simulink model "estimate_battery_soca"  (R2022a)
settings: Solver=VariableStepAuto  StartTime=0.0  StopTime=t_end  RelTol=1e-3
undefined symbols (not defined in the file): Bat_cap, eff_bcr, eff_id, eff_pcm, Np, Ns, OCV, Ri_cell, sigbuilder_block, SOC, SOC_init, V_ulim
settings Model: Creator=Geuk-Nam Kim  LastModifiedBy=ACL2022_13
settings SolverCC: ZeroCrossAlgorithm=Adaptive  AlgebraicLoopSolver=TrustRegion
settings DebuggingCC: IgnoredZcDiagnostic=none  UnconnectedInputMsg=warning  UnconnectedOutputMsg=warning  UnconnectedLineMsg=warning  SFMachineParentedDataDiag=warning

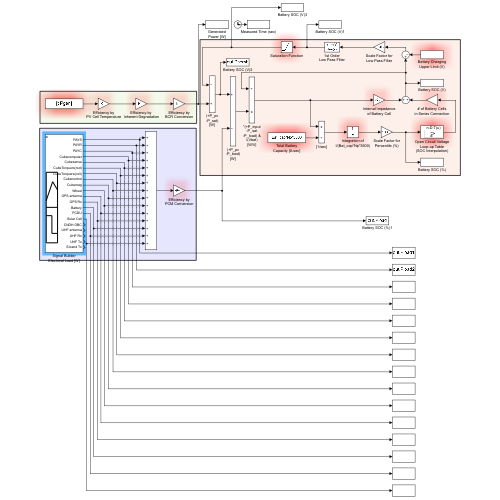
[thumbnail: Simulink's stored preview of the top-level diagram]
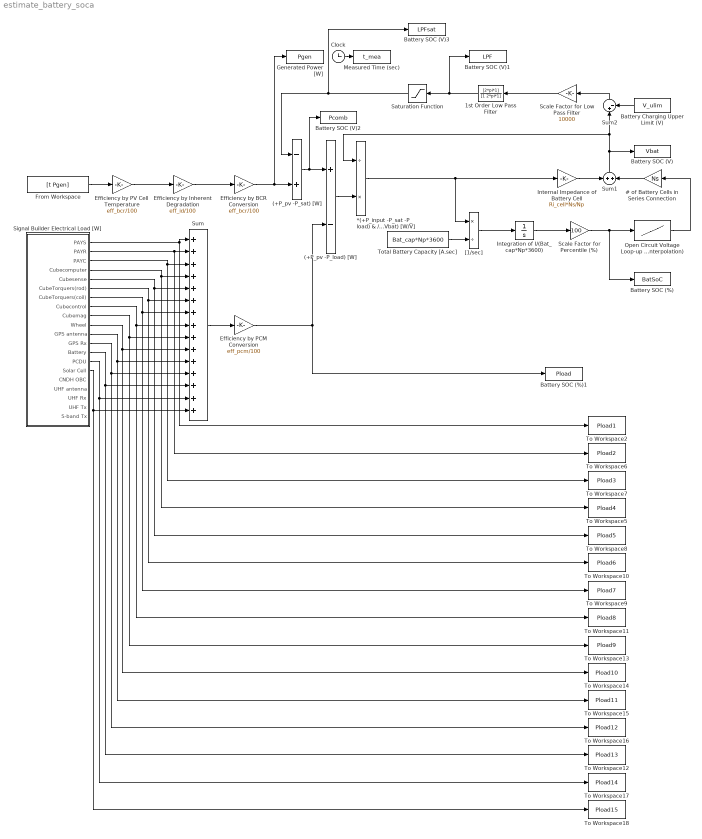
== system estimate_battery_soca ==
  # of Battery Cells in Series Connection : Gain  Gain=Ns
  (+P_pv -P_load) [W] : Sum  Inputs=+-
  (+P_pv -P_sat) [W] : Sum  Inputs=-+
  *(+P_input -P_sat -P_load) & /(Vbat) [W/V] : Product  Inputs=/*
  1st Order Low Pass Filter : TransferFcn  Numerator=[2*pi*1]  Denominator=[1 2*pi*1]
  Battery Charging Upper Limit (V) : Constant  Value=V_ulim
  Battery SOC (%) : ToWorkspace  VariableName=BatSoC  SampleTime=-1
  Battery SOC (%)1 : ToWorkspace  VariableName=Pload  SampleTime=-1
  Battery SOC (V) : ToWorkspace  VariableName=Vbat  SampleTime=-1
  Battery SOC (V)1 : ToWorkspace  VariableName=LPF  SampleTime=-1
  Battery SOC (V)2 : ToWorkspace  VariableName=Pcomb  SampleTime=-1
  Battery SOC (V)3 : ToWorkspace  VariableName=LPFsat  SampleTime=-1
  Clock : Clock
  "Efficiency by BCR Conversion " : Gain  Gain=eff_bcr/100
  Efficiency by PCM Conversion : Gain  Gain=eff_pcm/100
  Efficiency by PV Cell Temperature : Gain  Gain=eff_bcr/100
  Efficiency by Inherent Degradation : Gain  Gain=eff_id/100
  From Workspace : FromWorkspace  VariableName=[t Pgen]  SampleTime=-1
  Generated Power [W] : ToWorkspace  VariableName=Pgen  SampleTime=-1
  Integration of I/(Bat_cap*Np*3600) : Integrator  InitialCondition=SOC_init
  Internal Impedance of Battery Cell : Gain  Gain=Ri_cell*Ns/Np
  Measured Time (sec) : ToWorkspace  VariableName=t_mea  SampleTime=-1
  Open Circuit Voltage Loop-up Table (SOC Interpolation) : Lookup_n-D  NumberOfTableDimensions=1  BreakpointsForDimension1=SOC  Table=OCV  InternalRulePriority=Speed  RndMeth=Simplest
  Saturation Function : Saturate  UpperLimit=V_ulim  LowerLimit=0
  Scale Factor for Low Pass Filter : Gain  Gain=10000
  Scale Factor for Percentile (%) : Gain  Gain=100
  Signal Builder Electrical Load [W] : Subsystem  Tag=STV Subsys  LoadFcn=sigbuilder_block('load',[6 30 1428 680.25 ]);  StartFcn=sigbuilder_block('start');  StopFcn=sigbuilder_block('stop');  ClipboardFcn=sigbuilder_block('clipboard');  mask(Sigbuilder block){tuvar=[0:10]}
      mask help: Simulink:masks:SigbuilderBlock_MD
      mask init:
      | if ~strcmp(get_param(bdroot(gcbh),'SimulationStatus'),'stopped') tuvar = sigbuilder_block('maskInit'); end
      settings: CopyFcn=sigbuilder_block('copy');  DeleteFcn=sigbuilder_block('delete');  ModelCloseFcn=sigbuilder_block('modelClose');  PreSaveFcn=sigbuilder_block('preSave');  PauseFcn=sigbuilder_block('pause');  ContinueFcn=sigbuilder_block('continue');  NameChangeFcn=sigbuilder_block('namechange');  OpenFcn=sigbuilder_block('open',[6 30 1428 680.25 ]);  CloseFcn=sigbuilder_block('close');
      mask Display: plot(0, 0, 100, 100,[2, 2, 32, 32, 2], [68, 8, 8, 68, 68],[32, 2], [38, 38], [32, 19, 2],[53, 60, 44], [32, 17, 17, 2],[16, 16, 31, 31]);txt = getActiveGroup(gcbh);text(2, 100, txt,'verticalAlignment', 'top');
  Sum : Sum  Inputs=15
  Sum1 : Sum  Inputs=+|+
  Sum2 : Sum  Inputs=|+-
  To Workspace10 : ToWorkspace  VariableName=Pload6  SampleTime=-1
  To Workspace11 : ToWorkspace  VariableName=Pload8  SampleTime=-1
  To Workspace12 : ToWorkspace  VariableName=Pload13  SampleTime=-1
  To Workspace13 : ToWorkspace  VariableName=Pload9  SampleTime=-1
  To Workspace14 : ToWorkspace  VariableName=Pload10  SampleTime=-1
  To Workspace15 : ToWorkspace  VariableName=Pload11  SampleTime=-1
  To Workspace16 : ToWorkspace  VariableName=Pload12  SampleTime=-1
  To Workspace17 : ToWorkspace  VariableName=Pload14  SampleTime=-1
  To Workspace18 : ToWorkspace  VariableName=Pload15  SampleTime=-1
  To Workspace2 : ToWorkspace  VariableName=Pload1  SampleTime=-1
  To Workspace5 : ToWorkspace  VariableName=Pload4  SampleTime=-1
  To Workspace6 : ToWorkspace  VariableName=Pload2  SampleTime=-1
  To Workspace7 : ToWorkspace  VariableName=Pload3  SampleTime=-1
  To Workspace8 : ToWorkspace  VariableName=Pload5  SampleTime=-1
  To Workspace9 : ToWorkspace  VariableName=Pload7  SampleTime=-1
  Total Battery Capacity [A.sec] : Constant  Value=Bat_cap*Np*3600
  "[1/sec]" : Product  Inputs=*/
  wires:
  From Workspace/1 -> Efficiency by PV Cell Temperature/1
  Open Circuit Voltage Loop-up Table (SOC Interpolation)/1 -> # of Battery Cells in Series Connection/1
  Signal Builder Electrical Load [W]/8(Cubecontrol) -> To Workspace11/1, Sum/8
  Total Battery Capacity [A.sec]/1 -> "[1/sec]"/2
  Sum2/1 -> Scale Factor for Low Pass Filter/1
  "[1/sec]"/1 -> Integration of I/(Bat_cap*Np*3600)/1
  Scale Factor for Percentile (%)/1 -> Battery SOC (%)/1, Open Circuit Voltage Loop-up Table (SOC Interpolation)/1
  Signal Builder Electrical Load [W]/1(PAYS) -> Sum/1, To Workspace2/1
  "Efficiency by BCR Conversion "/1 -> (+P_pv -P_sat) [W]/2, Generated Power [W]/1
  Signal Builder Electrical Load [W]/14(PCDU) -> To Workspace17/1, Sum/14
  # of Battery Cells in Series Connection/1 -> Sum1/2
  Signal Builder Electrical Load [W]/4(Cubecomputer) -> To Workspace5/1, Sum/4
  Integration of I/(Bat_cap*Np*3600)/1 -> Scale Factor for Percentile (%)/1
  *(+P_input -P_sat -P_load) & /(Vbat) [W/V]/1 -> "[1/sec]"/1, Internal Impedance of Battery Cell/1
  Internal Impedance of Battery Cell/1 -> Sum1/1
  1st Order Low Pass Filter/1 -> Battery SOC (V)1/1, Saturation Function/1
  Signal Builder Electrical Load [W]/12(GPS Rx) -> To Workspace16/1, Sum/12
  Signal Builder Electrical Load [W]/13(Battery) -> To Workspace12/1, Sum/13
  Saturation Function/1 -> Battery SOC (V)3/1, (+P_pv -P_sat) [W]/1
  Signal Builder Electrical Load [W]/10(Wheel) -> To Workspace14/1, Sum/10
  (+P_pv -P_load) [W]/1 -> *(+P_input -P_sat -P_load) & /(Vbat) [W/V]/2
  Signal Builder Electrical Load [W]/11(GPS antenna) -> To Workspace15/1, Sum/11
  Signal Builder Electrical Load [W]/2(PAYR) -> To Workspace6/1, Sum/2
  Battery Charging Upper Limit (V)/1 -> Sum2/2
  Signal Builder Electrical Load [W]/15(Solar Cell) -> To Workspace18/1, Sum/15
  Signal Builder Electrical Load [W]/6(CubeTorquers(rod)) -> To Workspace10/1, Sum/6
  Sum1/1 -> Sum2/1, *(+P_input -P_sat -P_load) & /(Vbat) [W/V]/1, Battery SOC (V)/1
  Signal Builder Electrical Load [W]/5(Cubesense) -> To Workspace8/1, Sum/5
  Signal Builder Electrical Load [W]/9(Cubemag) -> To Workspace13/1, Sum/9
  Clock/1 -> Measured Time (sec)/1
  Efficiency by Inherent Degradation/1 -> "Efficiency by BCR Conversion "/1
  Sum/1 -> Efficiency by PCM Conversion/1
  Signal Builder Electrical Load [W]/3(PAYC) -> To Workspace7/1, Sum/3
  Efficiency by PV Cell Temperature/1 -> Efficiency by Inherent Degradation/1
  Signal Builder Electrical Load [W]/7(CubeTorquers(coil)) -> To Workspace9/1, Sum/7
  (+P_pv -P_sat) [W]/1 -> Battery SOC (V)2/1, (+P_pv -P_load) [W]/1
  Scale Factor for Low Pass Filter/1 -> 1st Order Low Pass Filter/1
  Efficiency by PCM Conversion/1 -> Battery SOC (%)1/1, (+P_pv -P_load) [W]/2

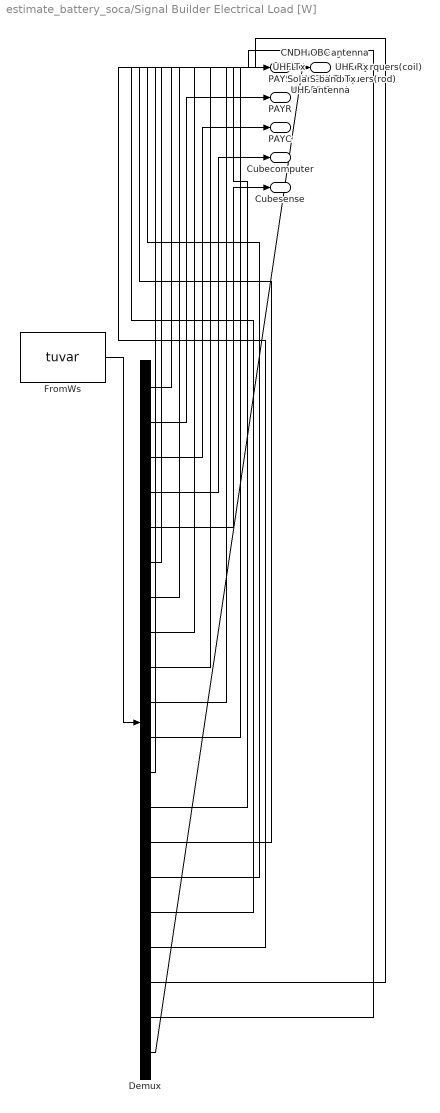
== system estimate_battery_soca/Signal Builder Electrical Load [W] ==
  Demux : Demux  Tag=STV Demux  Outputs=20
      settings: DisplayOption=none
  FromWs : FromWorkspace  Tag=STV FromWs  VariableName=tuvar
      SigBuilderData=|
      | common.afterFinalStr = 'Extrapolate'
      | common.sampleTime = '0'
      | dataSet(1).timeRange = [1 5678]
      | dataSet(1).name = 'a'
      | dataSet(2).timeRange = [1 5678]
      | dataSet(2).name = 'b'
      | dataSet(3).timeRange = [1 5678]
      | dataSet(3).name = 'c'
      | dataSet(4).timeRange = [1 5678]
      | dataSet(4).name = 'd'
      | sbobj.Name = 'Signal Builder'
      | sbobj.Groups(1).Name = 'a'
      | sbobj.Groups(1).Signals(1).Name = 'PAYS'
      | sbobj.Groups(1).Signals(1).XData = [1 2 3 4 5 6 7 8 9 10 11 12 ... (5678 elements, 1x5678)]
      | sbobj.Groups(1).Signals(1).YData = [0.2 0.2 0.2 0.2 0.2 0.2 0.2 0.2 0.2 0.2 0.2 0.2 ... (5678 elements, 1x5678)]
      | sbobj.Groups(1).Signals(2).Name = 'PAYR'
      | sbobj.Groups(1).Signals(2).XData = [1 2 3 4 5 6 7 8 9 10 11 12 ... (5678 elements, 1x5678)]
      | sbobj.Groups(1).Signals(2).YData = [0 0 0 0 0 0 0 0 0 0 0 0 ... (5678 elements, 1x5678)]
      | sbobj.Groups(1).Signals(3).Name = 'PAYC'
      | sbobj.Groups(1).Signals(3).XData = [1 2 3 4 5 6 7 8 9 10 11 12 ... (5678 elements, 1x5678)]
      | sbobj.Groups(1).Signals(3).YData = [1.3002 1.3002 1.3002 1.3002 1.3002 1.3002 1.3002 1.3002 1.3002 1.3002 1.3002 1.3002 ... (5678 elements, 1x5678)]
      | sbobj.Groups(1).Signals(4).Name = 'Cubecomputer'
      | sbobj.Groups(1).Signals(4).XData = [1 2 3 4 5 6 7 8 9 10 11 12 ... (5678 elements, 1x5678)]
      | sbobj.Groups(1).Signals(4).YData = [0.44 0.44 0.44 0.44 0.44 0.44 0.44 0.44 0.44 0.44 0.44 0.44 ... (5678 elements, 1x5678)]
      | sbobj.Groups(1).Signals(5).Name = 'Cubesense'
      | sbobj.Groups(1).Signals(5).XData = [1 2 3 4 5 6 7 8 9 10 11 12 ... (5678 elements, 1x5678)]
      | sbobj.Groups(1).Signals(5).YData = [0.8 0.8 0.8 0.8 0.8 0.8 0.8 0.8 0.8 0.8 0.8 0.8 ... (5678 elements, 1x5678)]
      | sbobj.Groups(1).Signals(6).Name = 'CubeTorquers(rod)'
      | sbobj.Groups(1).Signals(6).XData = [1 2 3 4 5 6 7 8 9 10 11 12 ... (5678 elements, 1x5678)]
      | sbobj.Groups(1).Signals(6).YData = [1.535 1.535 1.535 1.535 1.535 1.535 1.535 1.535 1.535 1.535 1.535 1.535 ... (5678 elements, 1x5678)]
      | sbobj.Groups(1).Signals(7).Name = 'CubeTorquers(coil)'
      | sbobj.Groups(1).Signals(7).XData = [1 2 3 4 5 6 7 8 9 10 11 12 ... (5678 elements, 1x5678)]
      | sbobj.Groups(1).Signals(7).YData = [0.192 0.192 0.192 0.192 0.192 0.192 0.192 0.192 0.192 0.192 0.192 0.192 ... (5678 elements, 1x5678)]
      | sbobj.Groups(1).Signals(8).Name = 'Cubecontrol'
      | sbobj.Groups(1).Signals(8).XData = [1 2 3 4 5 6 7 8 9 10 11 12 ... (5678 elements, 1x5678)]
      | sbobj.Groups(1).Signals(8).YData = [0.6 0.6 0.6 0.6 0.6 0.6 0.6 0.6 0.6 0.6 0.6 0.6 ... (5678 elements, 1x5678)]
      | sbobj.Groups(1).Signals(9).Name = 'Cubemag'
      | sbobj.Groups(1).Signals(9).XData = [1 2 3 4 5 6 7 8 9 10 11 12 ... (5678 elements, 1x5678)]
      | sbobj.Groups(1).Signals(9).YData = [0.105 0.105 0.105 0.105 0.105 0.105 0.105 0.105 0.105 0.105 0.105 0.105 ... (5678 elements, 1x5678)]
      | sbobj.Groups(1).Signals(10).Name = 'Wheel'
      | sbobj.Groups(1).Signals(10).XData = [1 2 3 4 5 6 7 8 9 10 11 12 ... (5678 elements, 1x5678)]
      | sbobj.Groups(1).Signals(10).YData = [8.04 8.04 8.04 8.04 8.04 8.04 8.04 8.04 8.04 8.04 8.04 8.04 ... (5678 elements, 1x5678)]
      | sbobj.Groups(1).Signals(11).Name = 'GPS antenna'
      | sbobj.Groups(1).Signals(11).XData = [1 2 3 4 5 6 7 8 9 10 11 12 ... (5678 elements, 1x5678)]
      | sbobj.Groups(1).Signals(11).YData = [0 0 0 0 0 0 0 0 0 0 0 0 ... (5678 elements, 1x5678)]
      | sbobj.Groups(1).Signals(12).Name = 'GPS Rx'
      | sbobj.Groups(1).Signals(12).XData = [1 2 3 4 5 6 7 8 9 10 11 12 ... (5678 elements, 1x5678)]
      | sbobj.Groups(1).Signals(12).YData = [3.9 3.9 3.9 3.9 3.9 3.9 3.9 3.9 3.9 3.9 3.9 3.9 ... (5678 elements, 1x5678)]
      | sbobj.Groups(1).Signals(13).Name = 'Battery'
      | sbobj.Groups(1).Signals(13).XData = [1 2 3 4 5 6 7 8 9 10 11 12 ... (5678 elements, 1x5678)]
      | sbobj.Groups(1).Signals(13).YData = [0.3 0.3 0.3 0.3 0.3 0.3 0.3 0.3 0.3 0.3 0.3 0.3 ... (5678 elements, 1x5678)]
      | sbobj.Groups(1).Signals(14).Name = 'PCDU'
      | sbobj.Groups(1).Signals(14).XData = [1 2 3 4 5 6 7 8 9 10 11 12 ... (5678 elements, 1x5678)]
      | sbobj.Groups(1).Signals(14).YData = [0.6 0.6 0.6 0.6 0.6 0.6 0.6 0.6 0.6 0.6 0.6 0.6 ... (5678 elements, 1x5678)]
      | sbobj.Groups(1).Signals(15).Name = 'Solar Cell'
      | sbobj.Groups(1).Signals(15).XData = [1 2 3 4 5 6 7 8 9 10 11 12 ... (5678 elements, 1x5678)]
      | sbobj.Groups(1).Signals(15).YData = [0 0 0 0 0 0 0 0 0 0 0 0 ... (5678 elements, 1x5678)]
      | sbobj.Groups(1).Signals(16).Name = 'CNDH OBC'
      | sbobj.Groups(1).Signals(16).XData = [1 2 3 4 5 6 7 8 9 10 11 12 ... (5678 elements, 1x5678)]
      | sbobj.Groups(1).Signals(16).YData = [1.85 1.85 1.85 1.85 1.85 1.85 1.85 1.85 1.85 1.85 1.85 1.85 ... (5678 elements, 1x5678)]
      | sbobj.Groups(1).Signals(17).Name = 'UHF antenna'
      | sbobj.Groups(1).Signals(17).XData = [1 2 3 4 5 6 7 8 9 10 11 12 ... (5678 elements, 1x5678)]
      | sbobj.Groups(1).Signals(17).YData = [0.04 0.04 0.04 0.04 0.04 0.04 0.04 0.04 0.04 0.04 0.04 0.04 ... (5678 elements, 1x5678)]
      | sbobj.Groups(1).Signals(18).Name = 'UHF Rx'
      | sbobj.Groups(1).Signals(18).XData = [1 2 3 4 5 6 7 8 9 10 11 12 ... (5678 elements, 1x5678)]
      | sbobj.Groups(1).Signals(18).YData = [1.0296 1.0296 1.0296 1.0296 1.0296 1.0296 1.0296 1.0296 1.0296 1.0296 1.0296 1.0296 ... (5678 elements, 1x5678)]
      | sbobj.Groups(1).Signals(19).Name = 'UHF Tx'
      | sbobj.Groups(1).Signals(19).XData = [1 2 3 4 5 6 7 8 9 10 11 12 ... (5678 elements, 1x5678)]
      | sbobj.Groups(1).Signals(19).YData = [1.32 1.32 1.32 1.32 1.32 1.32 1.32 1.32 1.32 1.32 1.32 1.32 ... (5678 elements, 1x5678)]
      | sbobj.Groups(1).Signals(20).Name = 'S-band Tx'
      | sbobj.Groups(1).Signals(20).XData = [1 2 3 4 5 6 7 8 9 10 11 12 ... (5678 elements, 1x5678)]
      | sbobj.Groups(1).Signals(20).YData = [0 0 0 0 0 0 0 0 0 0 0 0 ... (5678 elements, 1x5678)]
      | sbobj.Groups(1).TimeRange = [1 5678]
      | sbobj.Groups(2).Name = 'b'
      | sbobj.Groups(2).Signals(1).Name = 'PAYS'
      | sbobj.Groups(2).Signals(1).XData = [1 2 3 4 5 6 7 8 9 10 11 12 ... (5678 elements, 1x5678)]
      | sbobj.Groups(2).Signals(1).YData = [0 0 0 0 0 0 0 0 0 0 0 0 ... (5678 elements, 1x5678)]
      | sbobj.Groups(2).Signals(2).Name = 'PAYR'
      | sbobj.Groups(2).Signals(2).XData = [1 2 3 4 5 6 7 8 9 10 11 12 ... (5678 elements, 1x5678)]
      | sbobj.Groups(2).Signals(2).YData = [0 0 0 0 0 0 0 0 0 0 0 0 ... (5678 elements, 1x5678)]
      | sbobj.Groups(2).Signals(3).Name = 'PAYC'
      | sbobj.Groups(2).Signals(3).XData = [1 2 3 4 5 6 7 8 9 10 11 12 ... (5678 elements, 1x5678)]
      | sbobj.Groups(2).Signals(3).YData = [0 0 0 0 0 0 0 0 0 0 0 0 ... (5678 elements, 1x5678)]
      | sbobj.Groups(2).Signals(4).Name = 'Cubecomputer'
      | sbobj.Groups(2).Signals(4).XData = [1 2 3 4 5 6 7 8 9 10 11 12 ... (5678 elements, 1x5678)]
      | sbobj.Groups(2).Signals(4).YData = [0.44 0.44 0.44 0.44 0.44 0.44 0.44 0.44 0.44 0.44 0.44 0.44 ... (5678 elements, 1x5678)]
      | sbobj.Groups(2).Signals(5).Name = 'Cubesense'
      | sbobj.Groups(2).Signals(5).XData = [1 2 3 4 5 6 7 8 9 10 11 12 ... (5678 elements, 1x5678)]
      | sbobj.Groups(2).Signals(5).YData = [0.8 0.8 0.8 0.8 0.8 0.8 0.8 0.8 0.8 0.8 0.8 0.8 ... (5678 elements, 1x5678)]
      | sbobj.Groups(2).Signals(6).Name = 'CubeTorquers(rod)'
      | sbobj.Groups(2).Signals(6).XData = [1 2 3 4 5 6 7 8 9 10 11 12 ... (5678 elements, 1x5678)]
      | sbobj.Groups(2).Signals(6).YData = [1.535 1.535 1.535 1.535 1.535 1.535 1.535 1.535 1.535 1.535 1.535 1.535 ... (5678 elements, 1x5678)]
      | sbobj.Groups(2).Signals(7).Name = 'CubeTorquers(coil)'
      | sbobj.Groups(2).Signals(7).XData = [1 2 3 4 5 6 7 8 9 10 11 12 ... (5678 elements, 1x5678)]
      | sbobj.Groups(2).Signals(7).YData = [0.192 0.192 0.192 0.192 0.192 0.192 0.192 0.192 0.192 0.192 0.192 0.192 ... (5678 elements, 1x5678)]
      | sbobj.Groups(2).Signals(8).Name = 'Cubecontrol'
      | sbobj.Groups(2).Signals(8).XData = [1 2 3 4 5 6 7 8 9 10 11 12 ... (5678 elements, 1x5678)]
      | sbobj.Groups(2).Signals(8).YData = [0.6 0.6 0.6 0.6 0.6 0.6 0.6 0.6 0.6 0.6 0.6 0.6 ... (5678 elements, 1x5678)]
      | sbobj.Groups(2).Signals(9).Name = 'Cubemag'
      | sbobj.Groups(2).Signals(9).XData = [1 2 3 4 5 6 7 8 9 10 11 12 ... (5678 elements, 1x5678)]
      | sbobj.Groups(2).Signals(9).YData = [0.105 0.105 0.105 0.105 0.105 0.105 0.105 0.105 0.105 0.105 0.105 0.105 ... (5678 elements, 1x5678)]
      | sbobj.Groups(2).Signals(10).Name = 'Wheel'
      | sbobj.Groups(2).Signals(10).XData = [1 2 3 4 5 6 7 8 9 10 11 12 ... (5678 elements, 1x5678)]
      | sbobj.Groups(2).Signals(10).YData = [8.04 8.04 8.04 8.04 8.04 8.04 8.04 8.04 8.04 8.04 8.04 8.04 ... (5678 elements, 1x5678)]
      | sbobj.Groups(2).Signals(11).Name = 'GPS antenna'
      | sbobj.Groups(2).Signals(11).XData = [1 2 3 4 5 6 7 8 9 10 11 12 ... (5678 elements, 1x5678)]
      | sbobj.Groups(2).Signals(11).YData = [0 0 0 0 0 0 0 0 0 0 0 0 ... (5678 elements, 1x5678)]
      | sbobj.Groups(2).Signals(12).Name = 'GPS Rx'
      | sbobj.Groups(2).Signals(12).XData = [1 2 3 4 5 6 7 8 9 10 11 12 ... (5678 elements, 1x5678)]
      | sbobj.Groups(2).Signals(12).YData = [3.9 3.9 3.9 3.9 3.9 3.9 3.9 3.9 3.9 3.9 3.9 3.9 ... (5678 elements, 1x5678)]
      | sbobj.Groups(2).Signals(13).Name = 'Battery'
      | sbobj.Groups(2).Signals(13).XData = [1 2 3 4 5 6 7 8 9 10 11 12 ... (5678 elements, 1x5678)]
      | sbobj.Groups(2).Signals(13).YData = [0.3 0.3 0.3 0.3 0.3 0.3 0.3 0.3 0.3 0.3 0.3 0.3 ... (5678 elements, 1x5678)]
      | sbobj.Groups(2).Signals(14).Name = 'PCDU'
      | sbobj.Groups(2).Signals(14).XData = [1 2 3 4 5 6 7 8 9 10 11 12 ... (5678 elements, 1x5678)]
      | sbobj.Groups(2).Signals(14).YData = [0.6 0.6 0.6 0.6 0.6 0.6 0.6 0.6 0.6 0.6 0.6 0.6 ... (5678 elements, 1x5678)]
      | sbobj.Groups(2).Signals(15).Name = 'Solar Cell'
      | sbobj.Groups(2).Signals(15).XData = [1 2 3 4 5 6 7 8 9 10 11 12 ... (5678 elements, 1x5678)]
      | sbobj.Groups(2).Signals(15).YData = [0 0 0 0 0 0 0 0 0 0 0 0 ... (5678 elements, 1x5678)]
      | sbobj.Groups(2).Signals(16).Name = 'CNDH OBC'
      | sbobj.Groups(2).Signals(16).XData = [1 2 3 4 5 6 7 8 9 10 11 12 ... (5678 elements, 1x5678)]
      | sbobj.Groups(2).Signals(16).YData = [1.85 1.85 1.85 1.85 1.85 1.85 1.85 1.85 1.85 1.85 1.85 1.85 ... (5678 elements, 1x5678)]
      | sbobj.Groups(2).Signals(17).Name = 'UHF antenna'
      | sbobj.Groups(2).Signals(17).XData = [1 2 3 4 5 6 7 8 9 10 11 12 ... (5678 elements, 1x5678)]
      | sbobj.Groups(2).Signals(17).YData = [0 0 0 0 0 0 0 0 0 0 0 0 ... (5678 elements, 1x5678)]
      | sbobj.Groups(2).Signals(18).Name = 'UHF Rx'
      | sbobj.Groups(2).Signals(18).XData = [1 2 3 4 5 6 7 8 9 10 11 12 ... (5678 elements, 1x5678)]
      | sbobj.Groups(2).Signals(18).YData = [0.759 0.759 0.759 0.759 0.759 0.759 0.759 0.759 0.759 0.759 0.759 0.759 ... (5678 elements, 1x5678)]
      | sbobj.Groups(2).Signals(19).Name = 'UHF Tx'
      | sbobj.Groups(2).Signals(19).XData = [1 2 3 4 5 6 7 8 9 10 11 12 ... (5678 elements, 1x5678)]
      | sbobj.Groups(2).Signals(19).YData = [0 0 0 0 0 0 0 0 0 0 0 0 ... (5678 elements, 1x5678)]
      | sbobj.Groups(2).Signals(20).Name = 'S-band Tx'
      | sbobj.Groups(2).Signals(20).XData = [1 2 3 4 5 6 7 8 9 10 11 12 ... (5678 elements, 1x5678)]
      | sbobj.Groups(2).Signals(20).YData = [5 5 5 5 5 5 5 5 5 5 5 5 ... (5678 elements, 1x5678)]
      | sbobj.Groups(2).TimeRange = [1 5678]
      | sbobj.Groups(3).Name = 'c'
      | sbobj.Groups(3).Signals(1).Name = 'PAYS'
      | sbobj.Groups(3).Signals(1).XData = [1 2 3 4 5 6 7 8 9 10 11 12 ... (5678 elements, 1x5678)]
      | sbobj.Groups(3).Signals(1).YData = [0 0 0 0 0 0 0 0 0 0 0 0 ... (5678 elements, 1x5678)]
      | sbobj.Groups(3).Signals(2).Name = 'PAYR'
      | sbobj.Groups(3).Signals(2).XData = [1 2 3 4 5 6 7 8 9 10 11 12 ... (5678 elements, 1x5678)]
      | sbobj.Groups(3).Signals(2).YData = [0 0 0 0 0 0 0 0 0 0 0 0 ... (5678 elements, 1x5678)]
      | sbobj.Groups(3).Signals(3).Name = 'PAYC'
      | sbobj.Groups(3).Signals(3).XData = [1 2 3 4 5 6 7 8 9 10 11 12 ... (5678 elements, 1x5678)]
      | sbobj.Groups(3).Signals(3).YData = [0 0 0 0 0 0 0 0 0 0 0 0 ... (5678 elements, 1x5678)]
      | sbobj.Groups(3).Signals(4).Name = 'Cubecomputer'
      | sbobj.Groups(3).Signals(4).XData = [1 2 3 4 5 6 7 8 9 10 11 12 ... (5678 elements, 1x5678)]
      | sbobj.Groups(3).Signals(4).YData = [0.44 0.44 0.44 0.44 0.44 0.44 0.44 0.44 0.44 0.44 0.44 0.44 ... (5678 elements, 1x5678)]
      | sbobj.Groups(3).Signals(5).Name = 'Cubesense'
      | sbobj.Groups(3).Signals(5).XData = [1 2 3 4 5 6 7 8 9 10 11 12 ... (5678 elements, 1x5678)]
      | sbobj.Groups(3).Signals(5).YData = [0.8 0.8 0.8 0.8 0.8 0.8 0.8 0.8 0.8 0.8 0.8 0.8 ... (5678 elements, 1x5678)]
      | sbobj.Groups(3).Signals(6).Name = 'CubeTorquers(rod)'
      | sbobj.Groups(3).Signals(6).XData = [1 2 3 4 5 6 7 8 9 10 11 12 ... (5678 elements, 1x5678)]
      | sbobj.Groups(3).Signals(6).YData = [1.535 1.535 1.535 1.535 1.535 1.535 1.535 1.535 1.535 1.535 1.535 1.535 ... (5678 elements, 1x5678)]
      | sbobj.Groups(3).Signals(7).Name = 'CubeTorquers(coil)'
      | sbobj.Groups(3).Signals(7).XData = [1 2 3 4 5 6 7 8 9 10 11 12 ... (5678 elements, 1x5678)]
      | sbobj.Groups(3).Signals(7).YData = [0.192 0.192 0.192 0.192 0.192 0.192 0.192 0.192 0.192 0.192 0.192 0.192 ... (5678 elements, 1x5678)]
      | sbobj.Groups(3).Signals(8).Name = 'Cubecontrol'
      | sbobj.Groups(3).Signals(8).XData = [1 2 3 4 5 6 7 8 9 10 11 12 ... (5678 elements, 1x5678)]
      | sbobj.Groups(3).Signals(8).YData = [0.6 0.6 0.6 0.6 0.6 0.6 0.6 0.6 0.6 0.6 0.6 0.6 ... (5678 elements, 1x5678)]
      | sbobj.Groups(3).Signals(9).Name = 'Cubemag'
      | sbobj.Groups(3).Signals(9).XData = [1 2 3 4 5 6 7 8 9 10 11 12 ... (5678 elements, 1x5678)]
      | sbobj.Groups(3).Signals(9).YData = [0.105 0.105 0.105 0.105 0.105 0.105 0.105 0.105 0.105 0.105 0.105 0.105 ... (5678 elements, 1x5678)]
      | sbobj.Groups(3).Signals(10).Name = 'Wheel'
      | sbobj.Groups(3).Signals(10).XData = [1 2 3 4 5 6 7 8 9 10 11 12 ... (5678 elements, 1x5678)]
      | sbobj.Groups(3).Signals(10).YData = [8.04 8.04 8.04 8.04 8.04 8.04 8.04 8.04 8.04 8.04 8.04 8.04 ... (5678 elements, 1x5678)]
      | sbobj.Groups(3).Signals(11).Name = 'GPS antenna'
      | sbobj.Groups(3).Signals(11).XData = [1 2 3 4 5 6 7 8 9 10 11 12 ... (5678 elements, 1x5678)]
      | sbobj.Groups(3).Signals(11).YData = [0 0 0 0 0 0 0 0 0 0 0 0 ... (5678 elements, 1x5678)]
      | sbobj.Groups(3).Signals(12).Name = 'GPS Rx'
      | sbobj.Groups(3).Signals(12).XData = [1 2 3 4 5 6 7 8 9 10 11 12 ... (5678 elements, 1x5678)]
      | sbobj.Groups(3).Signals(12).YData = [3.9 3.9 3.9 3.9 3.9 3.9 3.9 3.9 3.9 3.9 3.9 3.9 ... (5678 elements, 1x5678)]
      | sbobj.Groups(3).Signals(13).Name = 'Battery'
      | sbobj.Groups(3).Signals(13).XData = [1 2 3 4 5 6 7 8 9 10 11 12 ... (5678 elements, 1x5678)]
      | sbobj.Groups(3).Signals(13).YData = [0.3 0.3 0.3 0.3 0.3 0.3 0.3 0.3 0.3 0.3 0.3 0.3 ... (5678 elements, 1x5678)]
      | sbobj.Groups(3).Signals(14).Name = 'PCDU'
      | sbobj.Groups(3).Signals(14).XData = [1 2 3 4 5 6 7 8 9 10 11 12 ... (5678 elements, 1x5678)]
      | sbobj.Groups(3).Signals(14).YData = [0.6 0.6 0.6 0.6 0.6 0.6 0.6 0.6 0.6 0.6 0.6 0.6 ... (5678 elements, 1x5678)]
      | sbobj.Groups(3).Signals(15).Name = 'Solar Cell'
      | sbobj.Groups(3).Signals(15).XData = [1 2 3 4 5 6 7 8 9 10 11 12 ... (5678 elements, 1x5678)]
      | sbobj.Groups(3).Signals(15).YData = [0 0 0 0 0 0 0 0 0 0 0 0 ... (5678 elements, 1x5678)]
      | sbobj.Groups(3).Signals(16).Name = 'CNDH OBC'
      | sbobj.Groups(3).Signals(16).XData = [1 2 3 4 5 6 7 8 9 10 11 12 ... (5678 elements, 1x5678)]
      | sbobj.Groups(3).Signals(16).YData = [1.85 1.85 1.85 1.85 1.85 1.85 1.85 1.85 1.85 1.85 1.85 1.85 ... (5678 elements, 1x5678)]
      | sbobj.Groups(3).Signals(17).Name = 'UHF antenna'
      | sbobj.Groups(3).Signals(17).XData = [1 2 3 4 5 6 7 8 9 10 11 12 ... (5678 elements, 1x5678)]
      | sbobj.Groups(3).Signals(17).YData = [0 0 0 0 0 0 0 0 0 0 0 0 ... (5678 elements, 1x5678)]
      | sbobj.Groups(3).Signals(18).Name = 'UHF Rx'
      | sbobj.Groups(3).Signals(18).XData = [1 2 3 4 5 6 7 8 9 10 11 12 ... (5678 elements, 1x5678)]
      | sbobj.Groups(3).Signals(18).YData = [0.759 0.759 0.759 0.759 0.759 0.759 0.759 0.759 0.759 0.759 0.759 0.759 ... (5678 elements, 1x5678)]
      | sbobj.Groups(3).Signals(19).Name = 'UHF Tx'
      | sbobj.Groups(3).Signals(19).XData = [1 2 3 4 5 6 7 8 9 10 11 12 ... (5678 elements, 1x5678)]
      | sbobj.Groups(3).Signals(19).YData = [0 0 0 0 0 0 0 0 0 0 0 0 ... (5678 elements, 1x5678)]
      | sbobj.Groups(3).Signals(20).Name = 'S-band Tx'
      | sbobj.Groups(3).Signals(20).XData = [1 2 3 4 5 6 7 8 9 10 11 12 ... (5678 elements, 1x5678)]
      | sbobj.Groups(3).Signals(20).YData = [5 5 5 5 5 5 5 5 5 5 5 5 ... (5678 elements, 1x5678)]
      | sbobj.Groups(3).TimeRange = [1 5678]
      | sbobj.Groups(4).Name = 'd'
      | sbobj.Groups(4).Signals(1).Name = 'PAYS'
      | sbobj.Groups(4).Signals(1).XData = [1 2 3 4 5 6 7 8 9 10 11 12 ... (5678 elements, 1x5678)]
      | sbobj.Groups(4).Signals(1).YData = [0 0 0 0 0 0 0 0 0 0 0 0 ... (5678 elements, 1x5678)]
      | sbobj.Groups(4).Signals(2).Name = 'PAYR'
      | sbobj.Groups(4).Signals(2).XData = [1 2 3 4 5 6 7 8 9 10 11 12 ... (5678 elements, 1x5678)]
      | sbobj.Groups(4).Signals(2).YData = [0 0 0 0 0 0 0 0 0 0 0 0 ... (5678 elements, 1x5678)]
      | sbobj.Groups(4).Signals(3).Name = 'PAYC'
      | sbobj.Groups(4).Signals(3).XData = [1 2 3 4 5 6 7 8 9 10 11 12 ... (5678 elements, 1x5678)]
      | sbobj.Groups(4).Signals(3).YData = [0 0 0 0 0 0 0 0 0 0 0 0 ... (5678 elements, 1x5678)]
      | sbobj.Groups(4).Signals(4).Name = 'Cubecomputer'
      | sbobj.Groups(4).Signals(4).XData = [1 2 3 4 5 6 7 8 9 10 11 12 ... (5678 elements, 1x5678)]
      | sbobj.Groups(4).Signals(4).YData = [0.24 0.24 0.24 0.24 0.24 0.24 0.24 0.24 0.24 0.24 0.24 0.24 ... (5678 elements, 1x5678)]
      | sbobj.Groups(4).Signals(5).Name = 'Cubesense'
      | sbobj.Groups(4).Signals(5).XData = [1 2 3 4 5 6 7 8 9 10 11 12 ... (5678 elements, 1x5678)]
      | sbobj.Groups(4).Signals(5).YData = [0.3 0.3 0.3 0.3 0.3 0.3 0.3 0.3 0.3 0.3 0.3 0.3 ... (5678 elements, 1x5678)]
      | sbobj.Groups(4).Signals(6).Name = 'CubeTorquers(rod)'
      | sbobj.Groups(4).Signals(6).XData = [1 2 3 4 5 6 7 8 9 10 11 12 ... (5678 elements, 1x5678)]
      | sbobj.Groups(4).Signals(6).YData = [0.07 0.07 0.07 0.07 0.07 0.07 0.07 0.07 0.07 0.07 0.07 0.07 ... (5678 elements, 1x5678)]
      | sbobj.Groups(4).Signals(7).Name = 'CubeTorquers(coil)'
      | sbobj.Groups(4).Signals(7).XData = [1 2 3 4 5 6 7 8 9 10 11 12 ... (5678 elements, 1x5678)]
      | sbobj.Groups(4).Signals(7).YData = [0.128 0.128 0.128 0.128 0.128 0.128 0.128 0.128 0.128 0.128 0.128 0.128 ... (5678 elements, 1x5678)]
      | sbobj.Groups(4).Signals(8).Name = 'Cubecontrol'
      | sbobj.Groups(4).Signals(8).XData = [1 2 3 4 5 6 7 8 9 10 11 12 ... (5678 elements, 1x5678)]
      | sbobj.Groups(4).Signals(8).YData = [0.4 0.4 0.4 0.4 0.4 0.4 0.4 0.4 0.4 0.4 0.4 0.4 ... (5678 elements, 1x5678)]
      | sbobj.Groups(4).Signals(9).Name = 'Cubemag'
      | sbobj.Groups(4).Signals(9).XData = [1 2 3 4 5 6 7 8 9 10 11 12 ... (5678 elements, 1x5678)]
      | sbobj.Groups(4).Signals(9).YData = [0.07 0.07 0.07 0.07 0.07 0.07 0.07 0.07 0.07 0.07 0.07 0.07 ... (5678 elements, 1x5678)]
      | sbobj.Groups(4).Signals(10).Name = 'Wheel'
      | sbobj.Groups(4).Signals(10).XData = [1 2 3 4 5 6 7 8 9 10 11 12 ... (5678 elements, 1x5678)]
      | sbobj.Groups(4).Signals(10).YData = [1.14 1.14 1.14 1.14 1.14 1.14 1.14 1.14 1.14 1.14 1.14 1.14 ... (5678 elements, 1x5678)]
      | sbobj.Groups(4).Signals(11).Name = 'GPS antenna'
      | sbobj.Groups(4).Signals(11).XData = [1 2 3 4 5 6 7 8 9 10 11 12 ... (5678 elements, 1x5678)]
      | sbobj.Groups(4).Signals(11).YData = [0 0 0 0 0 0 0 0 0 0 0 0 ... (5678 elements, 1x5678)]
      | sbobj.Groups(4).Signals(12).Name = 'GPS Rx'
      | sbobj.Groups(4).Signals(12).XData = [1 2 3 4 5 6 7 8 9 10 11 12 ... (5678 elements, 1x5678)]
      | sbobj.Groups(4).Signals(12).YData = [2.6 2.6 2.6 2.6 2.6 2.6 2.6 2.6 2.6 2.6 2.6 2.6 ... (5678 elements, 1x5678)]
      | sbobj.Groups(4).Signals(13).Name = 'Battery'
      | sbobj.Groups(4).Signals(13).XData = [1 2 3 4 5 6 7 8 9 10 11 12 ... (5678 elements, 1x5678)]
      | sbobj.Groups(4).Signals(13).YData = [0.2 0.2 0.2 0.2 0.2 0.2 0.2 0.2 0.2 0.2 0.2 0.2 ... (5678 elements, 1x5678)]
      | sbobj.Groups(4).Signals(14).Name = 'PCDU'
      | sbobj.Groups(4).Signals(14).XData = [1 2 3 4 5 6 7 8 9 10 11 12 ... (5678 elements, 1x5678)]
      | sbobj.Groups(4).Signals(14).YData = [0.4 0.4 0.4 0.4 0.4 0.4 0.4 0.4 0.4 0.4 0.4 0.4 ... (5678 elements, 1x5678)]
      | sbobj.Groups(4).Signals(15).Name = 'Solar Cell'
      | sbobj.Groups(4).Signals(15).XData = [1 2 3 4 5 6 7 8 9 10 11 12 ... (5678 elements, 1x5678)]
      | sbobj.Groups(4).Signals(15).YData = [0 0 0 0 0 0 0 0 0 0 0 0 ... (5678 elements, 1x5678)]
      | sbobj.Groups(4).Signals(16).Name = 'CNDH OBC'
      | sbobj.Groups(4).Signals(16).XData = [1 2 3 4 5 6 7 8 9 10 11 12 ... (5678 elements, 1x5678)]
      | sbobj.Groups(4).Signals(16).YData = [0.858 0.858 0.858 0.858 0.858 0.858 0.858 0.858 0.858 0.858 0.858 0.858 ... (5678 elements, 1x5678)]
      | sbobj.Groups(4).Signals(17).Name = 'UHF antenna'
      | sbobj.Groups(4).Signals(17).XData = [1 2 3 4 5 6 7 8 9 10 11 12 ... (5678 elements, 1x5678)]
      | sbobj.Groups(4).Signals(17).YData = [0 0 0 0 0 0 0 0 0 0 0 0 ... (5678 elements, 1x5678)]
      | sbobj.Groups(4).Signals(18).Name = 'UHF Rx'
      | sbobj.Groups(4).Signals(18).XData = [1 2 3 4 5 6 7 8 9 10 11 12 ... (5678 elements, 1x5678)]
      | sbobj.Groups(4).Signals(18).YData = [0.51975 0.51975 0.51975 0.51975 0.51975 0.51975 0.51975 0.51975 0.51975 0.51975 0.51975 0.51975 ... (5678 elements, 1x5678)]
      | sbobj.Groups(4).Signals(19).Name = 'UHF Tx'
      | sbobj.Groups(4).Signals(19).XData = [1 2 3 4 5 6 7 8 9 10 11 12 ... (5678 elements, 1x5678)]
      | sbobj.Groups(4).Signals(19).YData = [0 0 0 0 0 0 0 0 0 0 0 0 ... (5678 elements, 1x5678)]
      | sbobj.Groups(4).Signals(20).Name = 'S-band Tx'
      | sbobj.Groups(4).Signals(20).XData = [1 2 3 4 5 6 7 8 9 10 11 12 ... (5678 elements, 1x5678)]
      | sbobj.Groups(4).Signals(20).YData = [0 0 0 0 0 0 0 0 0 0 0 0 ... (5678 elements, 1x5678)]
      | sbobj.Groups(4).TimeRange = [1 5678]
  PAYS : Outport  VectorParamsAs1DForOutWhenUnconnected=off
  PAYR : Outport  Tag=STV Outport  Port=2  VectorParamsAs1DForOutWhenUnconnected=off
  PAYC : Outport  Tag=STV Outport  Port=3  VectorParamsAs1DForOutWhenUnconnected=off
  Cubecomputer : Outport  Tag=STV Outport  Port=4  VectorParamsAs1DForOutWhenUnconnected=off
  Cubesense : Outport  Tag=STV Outport  Port=5  VectorParamsAs1DForOutWhenUnconnected=off
  CubeTorquers(rod) : Outport  Tag=STV Outport  Port=6  VectorParamsAs1DForOutWhenUnconnected=off
  CubeTorquers(coil) : Outport  Tag=STV Outport  Port=7  VectorParamsAs1DForOutWhenUnconnected=off
  Cubecontrol : Outport  Tag=STV Outport  Port=8  VectorParamsAs1DForOutWhenUnconnected=off
  Cubemag : Outport  Tag=STV Outport  Port=9  VectorParamsAs1DForOutWhenUnconnected=off
  Wheel : Outport  Tag=STV Outport  Port=10  VectorParamsAs1DForOutWhenUnconnected=off
  GPS antenna : Outport  Tag=STV Outport  Port=11  VectorParamsAs1DForOutWhenUnconnected=off
  GPS Rx : Outport  Tag=STV Outport  Port=12  VectorParamsAs1DForOutWhenUnconnected=off
  Battery : Outport  Tag=STV Outport  Port=13
  PCDU : Outport  Tag=STV Outport  Port=14
  Solar Cell : Outport  Tag=STV Outport  Port=15
  CNDH OBC : Outport  Tag=STV Outport  Port=16
  UHF antenna : Outport  Tag=STV Outport  Port=17
  UHF Rx : Outport  Tag=STV Outport  Port=18
  UHF Tx : Outport  Tag=STV Outport  Port=19
  S-band Tx : Outport  Tag=STV Outport  Port=20
  wires:
  Demux/1 -> PAYS/1
  Demux/2 -> PAYR/1
  Demux/3 -> PAYC/1
  Demux/4 -> Cubecomputer/1
  Demux/5 -> Cubesense/1
  Demux/6 -> CubeTorquers(rod)/1
  Demux/7 -> CubeTorquers(coil)/1
  FromWs/1 -> Demux/1
  Demux/8 -> Cubecontrol/1
  Demux/9 -> Cubemag/1
  Demux/10 -> Wheel/1
  Demux/11 -> GPS antenna/1
  Demux/12 -> GPS Rx/1
  Demux/13 -> Battery/1
  Demux/14 -> PCDU/1
  Demux/15 -> Solar Cell/1
  Demux/16 -> CNDH OBC/1
  Demux/17 -> UHF antenna/1
  Demux/18 -> UHF Rx/1
  Demux/19 -> UHF Tx/1
  Demux/20 -> S-band Tx/1
